simulink library "unifier_obm"  (R2023a)
settings: Solver=VariableStepAuto  StartTime=0.0  StopTime=10.0  RelTol=1e-3
undefined symbols (not defined in the file): b, c, dp_DEP, dp_FUSE_FIN, dp_HTU, dp_VTAIL, dp_VTAIL_INDUCED, dp_WING_root, dp_WING_tip, I, m, S, vtail_nodes, wing_nodes, xyz_cg, xyz_DEP
libraries: sharedutil x7, aerolibtransform2 x4, sharedtransform x2, matrix_library x1, shared6dofsys x1, shared6dof x1, simulink x1
(part 1 of 2)
settings Model: Creator=Thomas  LastModifiedBy=Reggie Johanes
settings DebuggingCC: UnconnectedInputMsg=warning  UnconnectedOutputMsg=warning  UnconnectedLineMsg=warning
settings ModelReferenceCC: EnableRefExpFcnMdlSchedulingChecks=on
settings RTWCC: DLArmComputeVersion=19.05

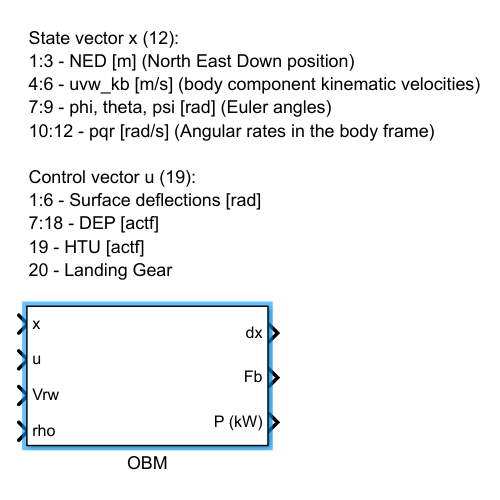
[thumbnail: Simulink's stored preview of the top-level diagram]
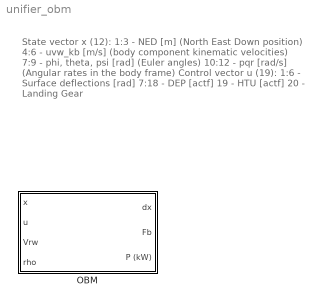
== system unifier_obm ==
  note: State vector x (12):
      | 1:3 - NED [m] (North East Down position)
      | 4:6 - uvw_kb [m/s] (body component kinematic velocities)
      | 7:9 - phi, theta, psi [rad] (Euler angles)
      | 10:12 - pqr [rad/s] (Angular rates in the body frame)
      |
      | Control vector u (19):
      | 1:6 - Surface deflections [rad]
      | 7:18 - DEP [actf]
      | 19 - HTU [actf]
      | 20 - Landing Gear
  OBM : Subsystem

== system unifier_obm/OBM ==
  x : Inport
  u : Inport  Port=2
  Vrw : Inport  Port=3
  rho : Inport  Port=4
  Aero : Subsystem
  Bus Selector : BusSelector  OutputSignals=Vrw,omegarw,Vrw_mag,beta,alpha,rho
  Cast{1,4,6..12} (9 alike) : DataTypeConversion  OutDataTypeStr=single  SaturateOnIntegerOverflow=off  RndMeth=Floor
  Demux : Demux  Outputs=[6,12,1,1]
  EOMandEnviroment : Subsystem
  Subsystems : Subsystem
  Sum : Sum  Inputs=|++
  Sum1 : Sum  Inputs=|++
  dx : Outport
  Fb : Outport  Port=2
  P (kW) : Outport  Port=3
  wires:
  Sum1/1 -> EOMandEnviroment/3(M)
  Cast1/1 -> Aero/8(u1 (rad))
  Subsystems/4(M) -> Sum1/2
  Subsystems/3(F) -> Sum/2
  Subsystems/2(u1_actual) -> Cast1/1
  Sum/1 -> Fb/1, EOMandEnviroment/2(F)
  Cast6/1 -> Aero/7(DEP_J)
  Subsystems/1(DEP_J) -> Cast6/1
  Aero/2(M) -> Sum1/1
  EOMandEnviroment/1(X2) -> Subsystems/1(X2)
  Aero/1(F) -> Sum/1
  u/1 -> Demux/1
  x/1 -> EOMandEnviroment/1(x)
  EOMandEnviroment/3(dx) -> dx/1
  Demux/1 -> Subsystems/3(u1 (rad))  "u1"
  Demux/2 -> Subsystems/4(u2 (actf))  "u2"
  Demux/3 -> Subsystems/5(u3 (actf))  "u3"
  rho/1 -> EOMandEnviroment/4(rho)
  Demux/4 -> Cast4/1  "u4"
  Subsystems/5(P) -> P (kW)/1
  Vrw/1 -> EOMandEnviroment/5(Vrw)
  Bus Selector/4 -> Cast11/1  "<beta>"
  Bus Selector/2 -> Cast9/1  "<omegarw>"
  Cast12/1 -> Aero/5(alpha)
  Bus Selector/6 -> Cast8/1  "<rho>"
  Cast11/1 -> Aero/4(beta)
  Bus Selector/3 -> Cast10/1  "<Vrw_mag>"
  Cast8/1 -> Aero/6(rho)
  Cast7/1 -> Aero/1(Vrw)
  Bus Selector/5 -> Cast12/1  "<alpha>"
  Cast10/1 -> Aero/3(Vrw_mag)
  EOMandEnviroment/2(X4) -> Subsystems/2(X4), Bus Selector/1
  Cast9/1 -> Aero/2(omegarw)
  Bus Selector/1 -> Cast7/1  "<Vrw>"
  Cast4/1 -> Aero/9(u4 (gear))

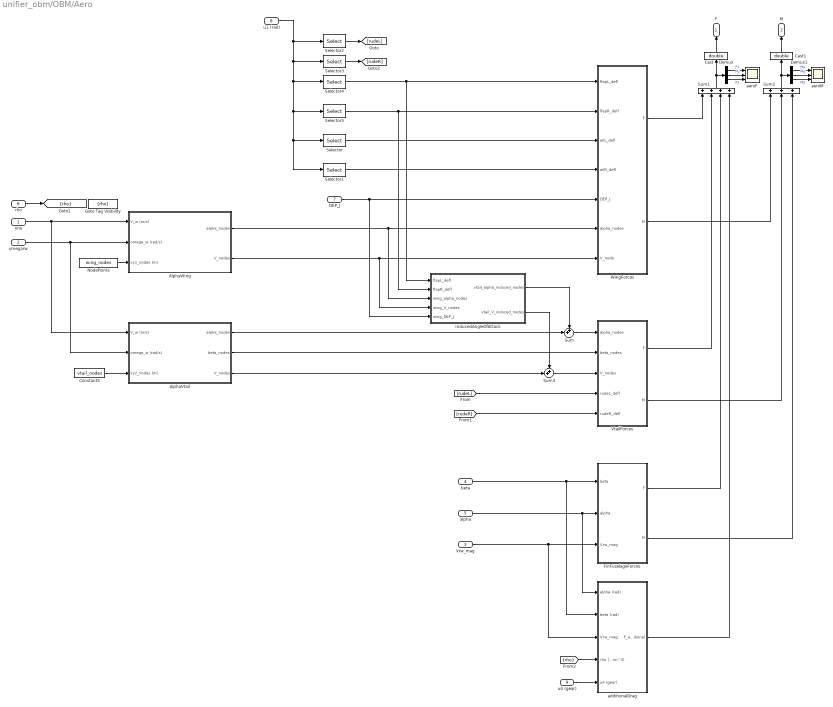
== system unifier_obm/OBM/Aero ==
  Vrw : Inport  OutDataTypeStr=single  Unit=m/s  PortDimensions=3  LockScale=on
  omegarw : Inport  Port=2  OutDataTypeStr=single  Unit=rad/s  PortDimensions=3  LockScale=on
  Vrw_mag : Inport  Port=3  OutDataTypeStr=single
  beta : Inport  Port=4  OutDataTypeStr=single
  alpha : Inport  Port=5  OutDataTypeStr=single
  rho : Inport  Port=6  OutDataTypeStr=single  Unit=kg/m^3  PortDimensions=1  LockScale=on
  DEP_J : Inport  Port=7  OutDataTypeStr=single  PortDimensions=12  LockScale=on
  u1 (rad) : Inport  Port=8
  u4 (gear) : Inport  Port=9
  AlphaVtail : Subsystem  TreatAsAtomicUnit=on
  AlphaWIng : Subsystem  TreatAsAtomicUnit=on
  Cast : DataTypeConversion  OutDataTypeStr=double  SaturateOnIntegerOverflow=off  RndMeth=Floor
  Cast1 : DataTypeConversion  OutDataTypeStr=double  SaturateOnIntegerOverflow=off  RndMeth=Floor
  Constant5 : Constant  Value=vtail_nodes
  Demux : Demux  Outputs=3
  Demux1 : Demux  Outputs=3
  FinFuselageForces : Subsystem
  Goto Tag Visibility : GotoTagVisibility  GotoTag=rho
  InducedAngleOfAttack : Subsystem
  NodePoints : Constant  Value=wing_nodes
  Selector : Selector  InputPortWidth=6  IndexOptions=Index vector (dialog)  Indices=1  OutputSizes=1
  Selector1 : Selector  InputPortWidth=6  IndexOptions=Index vector (dialog)  Indices=2  OutputSizes=1
  Selector2 : Selector  InputPortWidth=6  IndexOptions=Index vector (dialog)  Indices=3  OutputSizes=1
  Selector3 : Selector  InputPortWidth=6  IndexOptions=Index vector (dialog)  Indices=4  OutputSizes=1
  Selector4 : Selector  InputPortWidth=6  IndexOptions=Index vector (dialog)  Indices=5  OutputSizes=1
  Selector5 : Selector  InputPortWidth=6  IndexOptions=Index vector (dialog)  Indices=6  OutputSizes=1
  Sum : Sum  Inputs=++|
  Sum1 : Sum  Inputs=++++
  Sum2 : Sum  Inputs=+++
  Sum3 : Sum  Inputs=++|
  VtailForces : Subsystem
  WingForces : Subsystem
  additionalDrag : Subsystem
  aeroF : Scope  NumInputPorts=3
  aeroM : Scope  NumInputPorts=3
  F : Outport  Unit=N  PortDimensions=3  LockScale=on
  M : Outport  Port=2  Unit=N*m  PortDimensions=3  LockScale=on
  tag scope: rho=scoped
  wires:
  NodePoints/1 -> AlphaWIng/3(xyz_nodes (m))
  Constant5/1 -> AlphaVtail/3(xyz_nodes (m))
  Vrw/1 -> AlphaVtail/1(V_w (m/s)), AlphaWIng/1(V_w (m/s))
  omegarw/1 -> AlphaVtail/2(omega_w (rad/s)), AlphaWIng/2(omega_w (rad/s))
  AlphaWIng/2(V_nodes) -> WingForces/7(V_node), InducedAngleOfAttack/4(wing_V_nodes)
  DEP_J/1 -> WingForces/5(DEP_J), InducedAngleOfAttack/5(wing_DEP_J)
  Sum/1 -> VtailForces/1(alpha_nodes)
  rho/1 -> [rho]
  AlphaVtail/2(beta_nodes) -> VtailForces/2(beta_nodes)
  [rudeL] -> VtailForces/4(rudeL_defl)
  [rudeR] -> VtailForces/5(rudeR_defl)
  WingForces/1(F) -> Sum1/1
  VtailForces/1(F) -> Sum1/2
  WingForces/2(M) -> Sum2/1
  VtailForces/2(M) -> Sum2/2
  Sum1/1 -> Demux/1, Cast/1
  AlphaVtail/3(V_nodes) -> Sum3/2
  InducedAngleOfAttack/1(vtail_alpha_induced_nodes) -> Sum/1
  InducedAngleOfAttack/2(vtail_V_induced_nodes) -> Sum3/1
  Sum3/1 -> VtailForces/3(V_nodes)
  AlphaVtail/1(alpha_nodes) -> Sum/2
  Cast/1 -> F/1
  Cast1/1 -> M/1
  Vrw_mag/1 -> additionalDrag/3(Vrw_mag), FinFuselageForces/3(Vrw_mag)
  beta/1 -> additionalDrag/2(beta (rad)), FinFuselageForces/1(beta)
  FinFuselageForces/1(F) -> Sum1/3
  FinFuselageForces/2(M) -> Sum2/3
  Selector/1 -> WingForces/3(ailL_defl)
  Selector1/1 -> WingForces/4(ailR_defl)
  Selector4/1 -> WingForces/1(flapL_defl), InducedAngleOfAttack/1(flapL_defl)
  Selector5/1 -> WingForces/2(flapR_defl), InducedAngleOfAttack/2(flapR_defl)
  Selector2/1 -> [rudeL]
  Selector3/1 -> [rudeR]
  Demux/1 -> aeroF/1  "Fx"
  Demux/2 -> aeroF/2  "Fy"
  Demux/3 -> aeroF/3  "Fz"
  Sum2/1 -> Cast1/1, Demux1/1
  Demux1/2 -> aeroM/2  "My"
  Demux1/1 -> aeroM/1  "Mx"
  Demux1/3 -> aeroM/3  "Mz"
  AlphaWIng/1(alpha_nodes) -> WingForces/6(alpha_nodes), InducedAngleOfAttack/3(wing_alpha_nodes)
  alpha/1 -> additionalDrag/1(alpha (rad)), FinFuselageForces/2(alpha)
  [rho] -> additionalDrag/4(rho (kg/m^3))
  additionalDrag/1(F_additional) -> Sum1/4
  u4 (gear)/1 -> additionalDrag/5(u4 (gear))
  u1 (rad)/1 -> Selector1/1, Selector/1, Selector5/1, Selector4/1, Selector3/1, Selector2/1

== system unifier_obm/OBM/EOMandEnviroment ==
  note: State vector x (12):
      | 1:3 - NED [m] (North East Down position)
      | 4:6 - uvw_kb [m/s] (body component kinematic velocities)
      | 7:9 - phi, theta, psi [rad] (Euler angles)
      | 10:12 - pqr [rad/s] (Angular rates in the body frame)
  x : Inport
  F : Inport  Port=2
  M : Inport  Port=3
  rho : Inport  Port=4
  Vrw : Inport  Port=5
  Bus Creator : BusCreator  Inputs=8
  Conversion1 : Subsystem
  EOM : Subsystem  mask{mass=m, inertia=I}
      mask prompts: mass "Mass [kg]"; inertia "Inertia [kg/m^3]"
  Mux : Mux  Inputs=2
  Terminator : Terminator
  pqr : Selector  InputPortWidth=12  IndexOptions=Index vector (dialog)  Indices=10:12  OutputSizes=1
  X2 : Outport
  X4 : Outport  Port=2
  dx : Outport  Port=3
  wires:
  Conversion1/3(alpha) -> Bus Creator/5  "alpha"
  Bus Creator/1 -> X4/1
  Conversion1/4(beta) -> Bus Creator/6  "beta"
  Conversion1/1(Vrw_mag) -> Bus Creator/3  "Vrw_mag"
  pqr/1 -> Bus Creator/7, Mux/2  "omegarw"
  EOM/3(DCMbe) -> Bus Creator/1  "DCMbe"
  F/1 -> EOM/2(F)
  M/1 -> EOM/3(M)
  x/1 -> EOM/1(x), pqr/1
  EOM/1(dx) -> dx/1
  rho/1 -> Conversion1/2(rho), Bus Creator/8  "rho"
  Mux/1 -> X2/1
  EOM/2(Abe) -> Terminator/1
  Conversion1/2(Vrw_mag_eas) -> Bus Creator/4  "Vrw_mag_eas"
  Vrw/1 -> Bus Creator/2, Conversion1/1(Vrw), Mux/1  "Vrw"

== system unifier_obm/OBM/Subsystems ==
  X2 : Inport
  X4 : Inport  Port=2
  u1 (rad) : Inport  Port=3
  u2 (actf) : Inport  Port=4
  u3 (actf) : Inport  Port=5
  Actuators : Subsystem
  DEP1 : Subsystem
  Gravity : Subsystem
  HTU : Subsystem
  Sum : Sum  Inputs=+++
  Sum1 : Sum
  Sum2 : Sum  Inputs=|++
  DEP_J : Outport
  u1_actual : Outport  Port=2
  F : Outport  Port=3
  M : Outport  Port=4
  P : Outport  Port=5
  wires:
  X2/1 -> DEP1/1(X2)
  X4/1 -> HTU/2(X4), Gravity/1(X4), DEP1/2(X4)
  DEP1/1(DEP_J) -> DEP_J/1
  Sum/1 -> F/1
  Gravity/1(F) -> Sum/2
  HTU/1(F (N)) -> Sum/3
  Sum1/1 -> M/1
  HTU/2(M (Nm)) -> Sum1/2
  DEP1/2(F) -> Sum/1
  DEP1/3(M) -> Sum1/1
  u1 (rad)/1 -> Actuators/1(u1)
  Actuators/1(u1_actual) -> u1_actual/1
  u3 (actf)/1 -> HTU/1(u3 (actf))
  u2 (actf)/1 -> DEP1/3(u2 (actf))
  DEP1/4(P (kW)) -> Sum2/1
  HTU/3(P (kW)) -> Sum2/2
  Sum2/1 -> P/1

== system unifier_obm/OBM/Aero/AlphaVtail ==
  V_w (m/s) : Inport
  omega_w (rad/s) : Inport  Port=2
  xyz_nodes (m) : Inport  Port=3  Partition=on  PartitionDimension=2  PartitionWidth=1  PartitionOffset=0
  3x3 Cross Product : sharedutil/3x3 Cross Product  aMode=aMode
  Asin : Trigonometry  Operator=asin
  Atan : Trigonometry  Operator=atan
  Cast : DataTypeConversion  OutDataTypeStr=single  SaturateOnIntegerOverflow=off  RndMeth=Floor
  Constant : Constant  Value=xyz_cg
  Constant1 : Constant  Value=eps  OutDataTypeStr=single
  Demux : Demux  Outputs=3
  Divide : Product  Inputs=*/
  Divide1 : Product  Inputs=*/
  For Each : ForEach  DisableCoverage=on  SpecifiedNumIters=16
  Mux : Mux  Inputs=3
  Sum : Sum  Inputs=+-
  Sum1 : Sum  Inputs=++|
  Sum2 : Sum  Inputs=|++
  Sum3 : Sum  Inputs=|++
  V_inf : Fcn  Expr=sqrt(u(1)^2+u(2)^2+u(3)^2)
  alpha_nodes : Outport  ConcatenationDimension=2
  beta_nodes : Outport  Port=2  ConcatenationDimension=2
  V_nodes : Outport  Port=3  ConcatenationDimension=2
  wires:
  3x3 Cross Product/1 -> Sum1/1
  Sum/1 -> 3x3 Cross Product/1
  Constant/1 -> Cast/1
  xyz_nodes (m)/1 -> Sum/2
  omega_w (rad/s)/1 -> 3x3 Cross Product/2
  V_w (m/s)/1 -> Sum1/2
  Sum1/1 -> Demux/1
  Demux/1 -> Sum2/1, Mux/1  "u"
  Demux/3 -> Mux/3, Divide/1  "w"
  Divide/1 -> Atan/1
  Atan/1 -> alpha_nodes/1
  Sum2/1 -> Divide/2
  Constant1/1 -> Sum3/2, Sum2/2
  Divide1/1 -> Asin/1
  Demux/2 -> Mux/2, Divide1/1
  Mux/1 -> V_inf/1
  Asin/1 -> beta_nodes/1  "beta"
  V_inf/1 -> Sum3/1
  Sum3/1 -> V_nodes/1, Divide1/2
  Cast/1 -> Sum/1

== system unifier_obm/OBM/Aero/AlphaWIng ==
  V_w (m/s) : Inport
  omega_w (rad/s) : Inport  Port=2
  xyz_nodes (m) : Inport  Port=3  Partition=on  PartitionDimension=2  PartitionWidth=1  PartitionOffset=0
  Cast : DataTypeConversion  OutDataTypeStr=single  SaturateOnIntegerOverflow=off  RndMeth=Floor
  ComputeAlphaBetaV : Subsystem
  Constant : Constant  Value=xyz_cg
  Cross Product : matrix_library/Cross Product
  For Each : ForEach  DisableCoverage=on  SpecifiedNumIters=14
  Sum : Sum  Inputs=+-
  Sum1 : Sum  Inputs=++|
  Terminator : Terminator
  alpha_nodes : Outport  ConcatenationDimension=2
  V_nodes : Outport  Port=2  ConcatenationDimension=2
  wires:
  Cross Product/1 -> Sum1/1
  Sum/1 -> Cross Product/1
  Constant/1 -> Cast/1
  xyz_nodes (m)/1 -> Sum/2
  omega_w (rad/s)/1 -> Cross Product/2
  V_w (m/s)/1 -> Sum1/2
  Cast/1 -> Sum/1
  Sum1/1 -> ComputeAlphaBetaV/1(V_w_local)
  ComputeAlphaBetaV/3(V_nodes) -> V_nodes/1
  ComputeAlphaBetaV/2(beta_nodes) -> Terminator/1
  ComputeAlphaBetaV/1(alpha_nodes) -> alpha_nodes/1

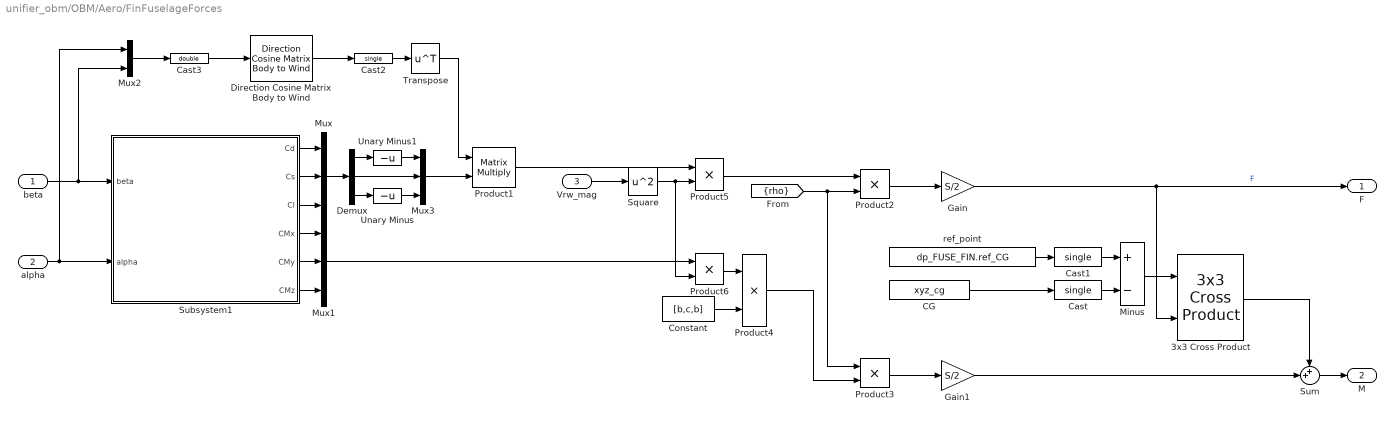
== system unifier_obm/OBM/Aero/FinFuselageForces ==
  beta : Inport
  alpha : Inport  Port=2
  Vrw_mag : Inport  Port=3  OutDataTypeStr=single
  3x3 Cross Product : sharedutil/3x3 Cross Product  aMode=aMode
  CG : Constant  Value=xyz_cg
  Cast : DataTypeConversion  OutDataTypeStr=single  SaturateOnIntegerOverflow=off  RndMeth=Floor
  Cast1 : DataTypeConversion  OutDataTypeStr=single  SaturateOnIntegerOverflow=off  RndMeth=Floor
  Cast2 : DataTypeConversion  OutDataTypeStr=single  SaturateOnIntegerOverflow=off  RndMeth=Floor
  Cast3 : DataTypeConversion  OutDataTypeStr=double  SaturateOnIntegerOverflow=off  RndMeth=Floor
  Constant : Constant  Value=[b,c,b]
  Demux : Demux  Outputs=3
  Direction Cosine Matrix Body to Wind : aerolibtransform2/Direction Cosine Matrix Body to Wind
  Gain : Gain  Gain=S/2
  Gain1 : Gain  Gain=S/2
  Minus : Sum  Inputs=+-
  Mux : Mux  Inputs=3
  Mux1 : Mux  Inputs=3
  Mux2 : Mux  Inputs=2
  Mux3 : Mux  Inputs=3
  Product1 : Product  Multiplication=Matrix(*)
  Product{2..6} (5 alike) : Product
  Square : Math  Operator=square
  Subsystem1 : Subsystem
  Sum : Sum  Inputs=++|
  Transpose : Math  Operator=transpose
  Unary Minus : UnaryMinus
  Unary Minus1 : UnaryMinus
  ref_point : Constant  Value=dp_FUSE_FIN.ref_CG
  F : Outport
  M : Outport  Port=2
  wires:
  Mux/1 -> Demux/1
  Product6/1 -> Product4/1
  Mux1/1 -> Product6/1
  Product5/1 -> Product2/1
  Vrw_mag/1 -> Square/1
  Product1/1 -> Product5/1
  Square/1 -> Product5/2, Product6/2
  Unary Minus1/1 -> Mux3/1
  Unary Minus/1 -> Mux3/3
  Mux3/1 -> Product1/2
  Demux/3 -> Unary Minus/1
  Demux/2 -> Mux3/2
  Demux/1 -> Unary Minus1/1
  Cast2/1 -> Transpose/1
  Cast3/1 -> Direction Cosine Matrix Body to Wind/1
  Direction Cosine Matrix Body to Wind/1 -> Cast2/1
  Transpose/1 -> Product1/1
  Mux2/1 -> Cast3/1
  Sum/1 -> M/1
  alpha/1 -> Subsystem1/2(alpha), Mux2/1
  beta/1 -> Subsystem1/1(beta), Mux2/2
  Cast1/1 -> Minus/1
  CG/1 -> Cast/1
  Minus/1 -> 3x3 Cross Product/1
  Cast/1 -> Minus/2
  ref_point/1 -> Cast1/1
  3x3 Cross Product/1 -> Sum/1
  Subsystem1/6(CMz) -> Mux1/3
  Subsystem1/5(CMy) -> Mux1/2
  Subsystem1/4(CMx) -> Mux1/1
  Subsystem1/3(Cl) -> Mux/3
  Subsystem1/2(Cs) -> Mux/2
  Subsystem1/1(Cd) -> Mux/1
  Product3/1 -> Gain1/1
  Gain/1 -> 3x3 Cross Product/2, F/1  "F"
  Constant/1 -> Product4/2
  [rho] -> Product3/1, Product2/2
  Gain1/1 -> Sum/2
  Product4/1 -> Product3/2
  Product2/1 -> Gain/1

== system unifier_obm/OBM/Aero/InducedAngleOfAttack ==
  flapL_defl : Inport
  flapR_defl : Inport  Port=2
  wing_alpha_nodes : Inport  Port=3  PortDimensions=14
  wing_V_nodes : Inport  Port=4  PortDimensions=14
  wing_DEP_J : Inport  Port=5  PortDimensions=12
  1-D Lookup Table : Lookup_n-D  NumberOfTableDimensions=1  BreakpointsForDimension1=wing_nodes(2,5:10)  BeginIndexSearchUsingPreviousIndexResult=on  TableSource=Input port  Table=tanh([-5:5])  ExtrapMethod=Clip  InternalRulePriority=Speed  RndMeth=Simplest
      settings: InputPortMap=u0,p221
  1-D Lookup Table1 : Lookup_n-D  NumberOfTableDimensions=1  BreakpointsForDimension1=wing_nodes(2,5:10)  BeginIndexSearchUsingPreviousIndexResult=on  TableSource=Input port  Table=tanh([-5:5])  ExtrapMethod=Clip  InternalRulePriority=Speed  RndMeth=Simplest
      settings: InputPortMap=u0,p221
  1-D Lookup Table2 : Lookup_n-D  NumberOfTableDimensions=1  BreakpointsForDimension1=wing_nodes(2,5:10)  BeginIndexSearchUsingPreviousIndexResult=on  TableSource=Input port  Table=tanh([-5:5])  ExtrapMethod=Clip  InternalRulePriority=Speed  RndMeth=Simplest
      settings: InputPortMap=u0,p221
  Constant : Constant  Value=ones(1,8)
  Constant1 : Constant  Value=ones(1,8)
  Constant7 : Constant  Value=vtail_nodes(2,:)
  Mux : Mux  Inputs=2
  Product : Product
  Product1 : Product
  Selector : Selector  InputPortWidth=14  IndexOptions=Index vector (dialog)  Indices=[5:10]  OutputSizes=1
  Selector1 : Selector  InputPortWidth=14  IndexOptions=Index vector (dialog)  Indices=[5:10]  OutputSizes=1
  Selector2 : Selector  InputPortWidth=12  IndexOptions=Index vector (dialog)  Indices=[4:9]  OutputSizes=1
  V_induced : Interpolation_n-D  NumberOfTableDimensions=5  Table=dp_VTAIL_INDUCED.V_induced  NumSelectionDims=1  InternalRulePriority=Speed  TableDataTypeStr=Inherit: Inherit from 'Table data'
      settings: InputPortMap=u0,u1,u2,u3,u4,u5,u6,u7,u8
  alpha_induced : Interpolation_n-D  NumberOfTableDimensions=5  Table=dp_VTAIL_INDUCED.alpha_induced  NumSelectionDims=1  InternalRulePriority=Speed  TableDataTypeStr=Inherit: Inherit from 'Table data'
      settings: InputPortMap=u0,u1,u2,u3,u4,u5,u6,u7,u8
  preLook : Subsystem
  vtail_alpha_induced_nodes : Outport  PortDimensions=16
  vtail_V_induced_nodes : Outport  Port=2  PortDimensions=16
  wires:
  1-D Lookup Table1/1 -> preLook/3(wing_V_inf)
  1-D Lookup Table2/1 -> preLook/4(wing_DEP_J)
  1-D Lookup Table/1 -> preLook/2(wing_alphas)
  Constant7/1 -> 1-D Lookup Table/1, 1-D Lookup Table2/1, 1-D Lookup Table1/1
  wing_V_nodes/1 -> Selector1/1
  wing_alpha_nodes/1 -> Selector/1
  preLook/1(Out1) -> alpha_induced/1, V_induced/1
  preLook/2(Out2) -> alpha_induced/2, V_induced/2
  preLook/3(Out8) -> alpha_induced/3, V_induced/3
  preLook/4(Out9) -> alpha_induced/4, V_induced/4
  preLook/5(Out3) -> alpha_induced/5, V_induced/5
  preLook/6(Out4) -> alpha_induced/6, V_induced/6
  preLook/7(Out6) -> alpha_induced/7, V_induced/7
  preLook/8(Out7) -> alpha_induced/8, V_induced/8
  preLook/9(Out5) -> alpha_induced/9, V_induced/9
  wing_DEP_J/1 -> Selector2/1
  flapL_defl/1 -> Product/2
  Constant/1 -> Product/1
  Constant1/1 -> Product1/1
  flapR_defl/1 -> Product1/2
  Product/1 -> Mux/1
  Product1/1 -> Mux/2
  Mux/1 -> preLook/1(wing_flap_defl)
  V_induced/1 -> vtail_V_induced_nodes/1
  alpha_induced/1 -> vtail_alpha_induced_nodes/1
  Selector/1 -> 1-D Lookup Table/2
  Selector1/1 -> 1-D Lookup Table1/2
  Selector2/1 -> 1-D Lookup Table2/2

== system unifier_obm/OBM/Aero/VtailForces ==
  alpha_nodes : Inport  PortDimensions=16
  beta_nodes : Inport  Port=2  PortDimensions=16
  V_nodes : Inport  Port=3  PortDimensions=16
  rudeL_defl : Inport  Port=4
  rudeR_defl : Inport  Port=5
  Constant : Constant  Value=ones(1,8)
  Constant1 : Constant  Value=ones(1,8)
  Matrix Concatenate1 : Concatenate  NumInputs=3  Mode=Multidimensional array  ConcatenateDimension=2
  Matrix Concatenate2 : Concatenate  NumInputs=3  Mode=Multidimensional array  ConcatenateDimension=2
  Mux : Mux  Inputs=2
  Product : Product
  Product1 : Product
  Reshape : Reshape
  Reshape1 : Reshape
  Subsystem : Subsystem
  Transpose : Math  Operator=transpose
  Transpose1 : Math  Operator=transpose
  VtailForces : Subsystem
  F : Outport
  M : Outport  Port=2
  wires:
  alpha_nodes/1 -> VtailForces/2(alpha_nodes)
  beta_nodes/1 -> VtailForces/3(beta_nodes)
  Product/1 -> Mux/1
  Product1/1 -> Mux/2
  Mux/1 -> VtailForces/1(rude_defl_nodes)
  Constant1/1 -> Product1/1
  Constant/1 -> Product/1
  rudeL_defl/1 -> Product/2
  rudeR_defl/1 -> Product1/2
  VtailForces/4(CMx) -> Matrix Concatenate2/1  "CMx"
  VtailForces/6(CMz) -> Matrix Concatenate2/3  "CMz"
  Matrix Concatenate2/1 -> Transpose1/1
  Subsystem/2(M) -> Reshape/1
  Transpose/1 -> Subsystem/2(F_matrix)
  Transpose1/1 -> Subsystem/3(M_matrix)
  VtailForces/2(Cy) -> Matrix Concatenate1/2  "CFy"
  VtailForces/5(CMy) -> Matrix Concatenate2/2  "CMy"
  VtailForces/1(Cx) -> Matrix Concatenate1/1  "CFx"
  Matrix Concatenate1/1 -> Transpose/1
  Subsystem/1(F) -> Reshape1/1
  VtailForces/3(Cz) -> Matrix Concatenate1/3  "CFz"
  V_nodes/1 -> Subsystem/1(V_nodes)
  Reshape/1 -> M/1
  Reshape1/1 -> F/1

== system unifier_obm/OBM/Aero/WingForces ==
  flapL_defl : Inport
  flapR_defl : Inport  Port=2
  ailL_defl : Inport  Port=3
  ailR_defl : Inport  Port=4
  DEP_J : Inport  Port=5  PortDimensions=12
  alpha_nodes : Inport  Port=6  PortDimensions=14
  V_node : Inport  Port=7  PortDimensions=14
  Demux : Demux  Outputs=3
  Demux1 : Demux  Outputs=3
  Left : Subsystem
  Mux : Mux  Inputs=3
  Mux1 : Mux  Inputs=3
  Reshape : Reshape
  Reshape1 : Reshape
  Right : Subsystem
  Subsystem : Subsystem
  Sum : Sum  Inputs=|++
  Sum1 : Sum  Inputs=|++
  Unary Minus : UnaryMinus
  Unary Minus1 : UnaryMinus
  Unary Minus2 : UnaryMinus
  F : Outport
  M : Outport  Port=2
  wires:
  ailL_defl/1 -> Left/2(aile_defl)
  flapL_defl/1 -> Left/1(flap_defl)
  ailR_defl/1 -> Right/2(aile_defl)
  DEP_J/1 -> Subsystem/1(DEP_J)
  flapR_defl/1 -> Right/1(flap_defl)
  alpha_nodes/1 -> Subsystem/2(alpha_nodes)
  V_node/1 -> Subsystem/3(V_nodes)
  Subsystem/1(DEP_J_Left) -> Left/3(DEP_J)
  Subsystem/2(alpha_nodes_Left) -> Left/4(alpha)
  Subsystem/3(V_nodes_Left) -> Left/5(V_node)
  Left/1(F) -> Demux/1
  Left/2(M) -> Demux1/1
  Demux/2 -> Unary Minus/1
  Demux1/1 -> Unary Minus1/1
  Demux1/3 -> Unary Minus2/1
  Demux1/2 -> Mux/2
  Unary Minus1/1 -> Mux/1
  Unary Minus2/1 -> Mux/3
  Unary Minus/1 -> Mux1/2
  Demux/1 -> Mux1/1
  Demux/3 -> Mux1/3
  Mux1/1 -> Sum/1
  Sum/1 -> F/1
  Mux/1 -> Sum1/1
  Sum1/1 -> M/1
  Right/1(F) -> Reshape/1
  Right/2(M) -> Reshape1/1
  Subsystem/5(alpha_nodes_Right) -> Right/4(alpha)
  Subsystem/6(V_nodes_Right) -> Right/5(V_node)
  Subsystem/4(DEP_J_Right) -> Right/3(DEP_J)
  Reshape/1 -> Sum/2
  Reshape1/1 -> Sum1/2

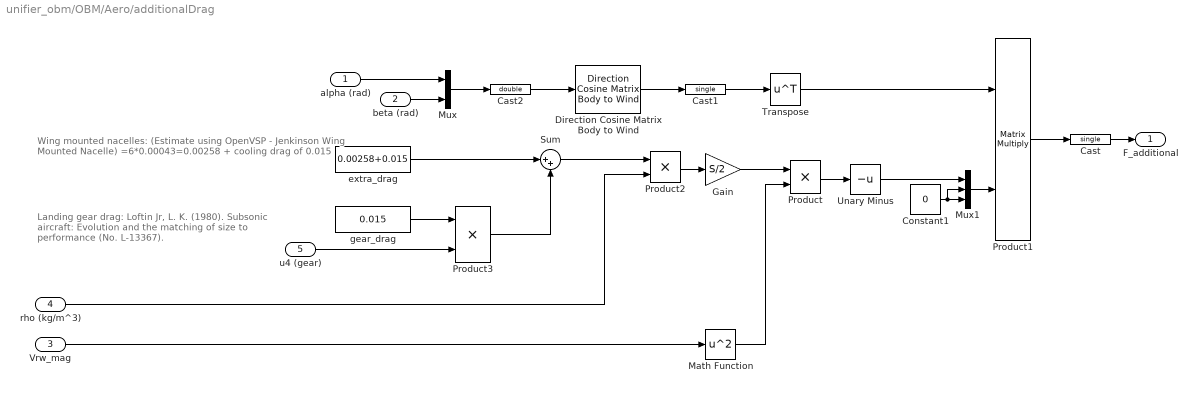
== system unifier_obm/OBM/Aero/additionalDrag ==
  note: Landing gear drag:
      | Loftin Jr, L. K. (1980). Subsonic aircraft: Evolution and the matching of size to performance (No. L-13367).
  note: Wing mounted nacelles:
      | (Estimate using OpenVSP - Jenkinson Wing Mounted Nacelle)
      | =6*0.00043=0.00258
      | + cooling drag of 0.015
  alpha (rad) : Inport
  beta (rad) : Inport  Port=2
  Vrw_mag : Inport  Port=3
  rho (kg/m^3) : Inport  Port=4
  u4 (gear) : Inport  Port=5
  Cast : DataTypeConversion  OutDataTypeStr=single  SaturateOnIntegerOverflow=off  RndMeth=Floor
  Cast1 : DataTypeConversion  OutDataTypeStr=single  SaturateOnIntegerOverflow=off  RndMeth=Floor
  Cast2 : DataTypeConversion  OutDataTypeStr=double  SaturateOnIntegerOverflow=off  RndMeth=Floor
  Constant1 : Constant  Value=0  OutDataTypeStr=single
  Direction Cosine Matrix Body to Wind : aerolibtransform2/Direction Cosine Matrix Body to Wind
  Gain : Gain  Gain=S/2
  Math Function : Math  Operator=square
  Mux : Mux  Inputs=2
  Mux1 : Mux  Inputs=3
  Product : Product  OutDataTypeStr=single
  Product1 : Product  Multiplication=Matrix(*)
  Product2 : Product
  Product3 : Product
  Sum : Sum  Inputs=|++
  Transpose : Math  Operator=transpose
  Unary Minus : UnaryMinus
  extra_drag : Constant  Value=0.00258+0.015  OutDataTypeStr=single
  gear_drag : Constant  Value=0.015  OutDataTypeStr=single
  F_additional : Outport
  wires:
  alpha (rad)/1 -> Mux/1
  Math Function/1 -> Product/2
  Product/1 -> Unary Minus/1
  Gain/1 -> Product/1
  Product2/1 -> Gain/1
  extra_drag/1 -> Sum/1
  Vrw_mag/1 -> Math Function/1
  rho (kg/m^3)/1 -> Product2/2
  Direction Cosine Matrix Body to Wind/1 -> Cast1/1
  Mux/1 -> Cast2/1
  beta (rad)/1 -> Mux/2
  Unary Minus/1 -> Mux1/1
  Transpose/1 -> Product1/1
  Mux1/1 -> Product1/2
  Constant1/1 -> Mux1/2, Mux1/3
  Product1/1 -> Cast/1
  Cast/1 -> F_additional/1
  Cast1/1 -> Transpose/1
  Cast2/1 -> Direction Cosine Matrix Body to Wind/1
  u4 (gear)/1 -> Product3/2
  gear_drag/1 -> Product3/1
  Sum/1 -> Product2/1
  Product3/1 -> Sum/2

== system unifier_obm/OBM/EOMandEnviroment/Conversion1 ==
  Vrw : Inport
  rho : Inport  Port=2
  Add : Sum
  Constant1 : Constant  Value=eps
  Demux3 : Demux  Outputs=3
  Divide1 : Product  Inputs=*/
  Dot Product : DotProduct  OutDataTypeStr=Inherit: Inherit via internal rule
  Gain : Gain  Gain=1/1.225
  Product : Product
  Sqrt : Sqrt
  Sqrt1 : Sqrt
  Trigonometric Function : Trigonometry  Operator=atan2
  Trigonometric Function1 : Trigonometry  Operator=asin
  Vrw_mag : Outport
  Vrw_mag_eas : Outport  Port=2
  alpha : Outport  Port=3
  beta : Outport  Port=4
  wires:
  Demux3/2 -> Divide1/1
  Constant1/1 -> Add/2
  Sqrt/1 -> Add/1
  Divide1/1 -> Trigonometric Function1/1
  Vrw/1 -> Dot Product/1, Dot Product/2, Demux3/1  "V_w"
  Demux3/3 -> Trigonometric Function/1
  Dot Product/1 -> Sqrt/1
  Demux3/1 -> Trigonometric Function/2
  Trigonometric Function1/1 -> beta/1  "beta"
  Trigonometric Function/1 -> alpha/1  "alpha"
  rho/1 -> Gain/1
  Gain/1 -> Sqrt1/1
  Sqrt1/1 -> Product/2
  Product/1 -> Vrw_mag_eas/1
  Add/1 -> Vrw_mag/1, Product/1, Divide1/2

== system unifier_obm/OBM/EOMandEnviroment/EOM ==
  note: Linear acceleration
  note: Euler_dot
  note: pqr_dot
  note: DCM, NED_dot
  x : Inport
  F : Inport  Port=2
  M : Inport  Port=3
  Calculate omega_dot : shared6dofsys/Calculate omega_dot  aMode=aMode
  Constant : Constant  Value=mass
  Constant1 : Constant  Value=inertia
  Constant2 : Constant  Value=zeros(3)
  Demux : Demux  Outputs=[3, 3, 3, 3]
  Mux6 : Mux
  Product : Product  Inputs=*/  SaturateOnIntegerOverflow=on  OutDataTypeStr=Inherit: Same as first input
  Rotation Angles to Direction Cosine Matrix : sharedtransform/Rotation Angles to Direction Cosine Matrix  rotationOrder=ZYX  aMode=aMode
  Selector : Selector  InputPortWidth=3  IndexOptions=Index vector (dialog)  Indices=[3 2 1]  OutputSizes=1
  Subsystem : Subsystem
  Sum : Sum  Inputs=|++  SaturateOnIntegerOverflow=on
  Terminator : Terminator
  Transpose : Math  Operator=transpose  SignedPower=on
  Vbxw : sharedutil/3x3 Cross Product  aMode=aMode
  Vector Concatenate : Concatenate  Mode=Multidimensional array
  "transform to Inertial axes " : shared6dof/6DOF (Euler Angles)/transform to Inertial axes   SystemSampleTime=-1  VariantActivationTime=update diagram  Latency=0  AutoFrameSizeCalculation=off
  dx : Outport
  Abe : Outport  Port=2
  DCMbe : Outport  Port=3
  wires:
  x/1 -> Demux/1
  Transpose/1 -> "transform to Inertial axes "/2
  F/1 -> Product/1
  Vbxw/1 -> Sum/2
  "transform to Inertial axes "/1 -> Mux6/1  "Ve"
  Sum/1 -> Mux6/2  "Abb"
  Product/1 -> Abe/1, Sum/1  "Abe"
  Vector Concatenate/1 -> Calculate omega_dot/2
  M/1 -> Calculate omega_dot/3
  Constant1/1 -> Vector Concatenate/1
  Subsystem/1(phidot thetadot psidot) -> Mux6/3
  Mux6/1 -> dx/1
  Demux/4 -> Subsystem/1(p q r), Calculate omega_dot/1, Vbxw/2  "pqr"
  Rotation Angles to Direction Cosine Matrix/1 -> DCMbe/1, Transpose/1  "DCMbe"
  Constant/1 -> Product/2
  Selector/1 -> Rotation Angles to Direction Cosine Matrix/1
  Demux/3 -> Subsystem/2(phi theta psi), Selector/1  "phithepsi"
  Calculate omega_dot/1 -> Mux6/4
  Constant2/1 -> Vector Concatenate/2
  Demux/2 -> Vbxw/1, "transform to Inertial axes "/1  "uvw_kb"
  Demux/1 -> Terminator/1  "NED"

== system unifier_obm/OBM/Subsystems/Actuators ==
  u1 : Inport
  Demux : Demux  Outputs=6
  Mux : Mux  Inputs=6
  Saturation : Saturate  UpperLimit=deg2rad(25)  LowerLimit=deg2rad(-25)
  Saturation1 : Saturate  UpperLimit=deg2rad(25)  LowerLimit=deg2rad(-25)
  Saturation2 : Saturate  UpperLimit=deg2rad(30)  LowerLimit=deg2rad(-30)
  Saturation3 : Saturate  UpperLimit=deg2rad(30)  LowerLimit=deg2rad(-30)
  Saturation4 : Saturate  UpperLimit=deg2rad(25)  LowerLimit=0
  Saturation6 : Saturate  UpperLimit=deg2rad(25)  LowerLimit=0
  u1_actual : Outport
  wires:
  u1/1 -> Demux/1
  Demux/1 -> Saturation/1
  Demux/2 -> Saturation1/1
  Demux/3 -> Saturation2/1
  Demux/4 -> Saturation3/1
  Saturation3/1 -> Mux/4
  Saturation2/1 -> Mux/3
  Saturation1/1 -> Mux/2
  Saturation/1 -> Mux/1
  Mux/1 -> u1_actual/1
  Demux/5 -> Saturation6/1
  Demux/6 -> Saturation4/1
  Saturation6/1 -> Mux/5
  Saturation4/1 -> Mux/6

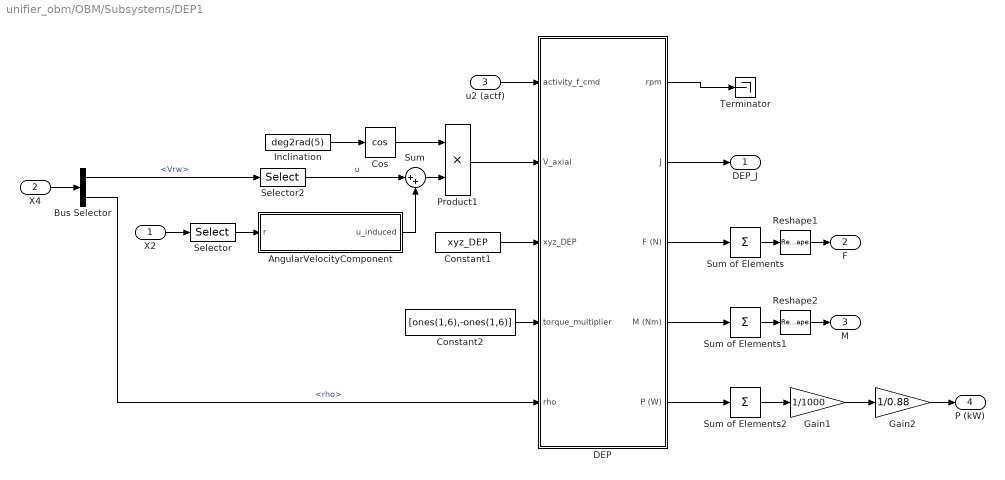
== system unifier_obm/OBM/Subsystems/DEP1 ==
  X2 : Inport
  X4 : Inport  Port=2
  u2 (actf) : Inport  Port=3
  AngularVelocityComponent : Subsystem
  Bus Selector : BusSelector  OutputSignals=Vrw,rho
  Constant1 : Constant  Value=xyz_DEP
  Constant2 : Constant  Value=[ones(1,6),-ones(1,6)]
  Cos : Trigonometry  Operator=cos
  DEP : Subsystem  TreatAsAtomicUnit=on
  Gain1 : Gain  Gain=1/1000
  Gain2 : Gain  Gain=1/0.88
  Inclination : Constant  Value=deg2rad(5)
  Product1 : Product
  Reshape1 : Reshape
  Reshape2 : Reshape
  Selector : Selector  InputPortWidth=6  IndexOptions=Index vector (dialog)  Indices=6  OutputSizes=1
  Selector2 : Selector  InputPortWidth=3  IndexOptions=Index vector (dialog)  Indices=1  OutputSizes=1
  Sum : Sum  Inputs=|++
  Sum of Elements : Sum  Inputs=+  CollapseMode=Specified dimension  CollapseDim=2
  Sum of Elements1 : Sum  Inputs=+  CollapseMode=Specified dimension  CollapseDim=2
  Sum of Elements2 : Sum  Inputs=+  CollapseMode=Specified dimension
  Terminator : Terminator
  DEP_J : Outport
  F : Outport  Port=2
  M : Outport  Port=3
  P (kW) : Outport  Port=4
  wires:
  X2/1 -> Selector/1
  X4/1 -> Bus Selector/1
  Bus Selector/1 -> Selector2/1  "<Vrw>"
  Product1/1 -> DEP/2(V_axial)
  u2 (actf)/1 -> DEP/1(activity_f_cmd)
  DEP/3(F (N)) -> Sum of Elements/1
  DEP/4(M (Nm)) -> Sum of Elements1/1
  Sum of Elements/1 -> Reshape1/1
  Sum of Elements1/1 -> Reshape2/1
  Reshape1/1 -> F/1
  Reshape2/1 -> M/1
  Constant1/1 -> DEP/3(xyz_DEP)
  Constant2/1 -> DEP/4(torque_multiplier)
  Bus Selector/2 -> DEP/5(rho)  "<rho>"
  DEP/2(J) -> DEP_J/1
  DEP/5(P (W)) -> Sum of Elements2/1
  Sum of Elements2/1 -> Gain1/1
  Selector2/1 -> Sum/1  "u"
  Inclination/1 -> Cos/1
  Cos/1 -> Product1/1
  Sum/1 -> Product1/2
  Gain1/1 -> Gain2/1
  Gain2/1 -> P (kW)/1
  Selector/1 -> AngularVelocityComponent/1(r)
  AngularVelocityComponent/1(u_induced) -> Sum/2
  DEP/1(rpm) -> Terminator/1

== system unifier_obm/OBM/Subsystems/Gravity ==
  X4 : Inport
  Bus Selector : BusSelector  OutputSignals=DCMbe
  Constant : Constant  Value=0
  Constant1 : Constant  Value=m
  Multiply : Gain  Gain=9.80665
  Mux : Mux  Inputs=3
  Product : Product  Multiplication=Matrix(*)
  F : Outport
  wires:
  Product/1 -> F/1  "F"
  Bus Selector/1 -> Product/1  "<DCMbe>"
  X4/1 -> Bus Selector/1
  Multiply/1 -> Mux/3
  Constant/1 -> Mux/2, Mux/1
  Mux/1 -> Product/2
  Constant1/1 -> Multiply/1

== system unifier_obm/OBM/Subsystems/HTU ==
  u3 (actf) : Inport
  X4 : Inport  Port=2
  1-D Lookup Table1 : Lookup_n-D  NumberOfTableDimensions=1  BreakpointsForDimension1=[-0.5,1.5]  IndexSearchMethod=Linear search  BeginIndexSearchUsingPreviousIndexResult=on  Table=[-5000, 15000]  ExtrapMethod=Clip  InternalRulePriority=Speed  RndMeth=Simplest
  Bus Selector : BusSelector  OutputSignals=Vrw_mag_eas
  Constant : Constant  Value=0
  Gain : Gain  Gain=1/0.92
  Mux : Mux  Inputs=3
  Mux1 : Mux  Inputs=3
  PropAndMotor : Subsystem
  F (N) : Outport
  M (Nm) : Outport  Port=2
  P (kW) : Outport  Port=3
  wires:
  Mux1/1 -> M (Nm)/1
  Constant/1 -> Mux1/2, Mux1/3, Mux1/1, Mux/3, Mux/2
  Mux/1 -> F (N)/1
  PropAndMotor/2(T (N)) -> Mux/1
  PropAndMotor/1(P (kW)) -> Gain/1
  X4/1 -> Bus Selector/1
  1-D Lookup Table1/1 -> PropAndMotor/2(T_cmd (N))
  Bus Selector/1 -> PropAndMotor/1(Vrw_mag_eas)  "<Vrw_mag_eas>"
  u3 (actf)/1 -> 1-D Lookup Table1/1
  Gain/1 -> P (kW)/1

== system unifier_obm/OBM/Aero/AlphaWIng/ComputeAlphaBetaV ==
  V_w_local : Inport
  Asin : Trigonometry  Operator=asin
  Atan : Trigonometry  Operator=atan
  Constant1 : Constant  Value=eps  OutDataTypeStr=single
  Demux : Demux  Outputs=3
  Divide : Product  Inputs=*/
  Divide1 : Product  Inputs=*/
  Dot Product : DotProduct  OutDataTypeStr=Inherit: Inherit via internal rule
  Square Root : Sqrt
  Sum2 : Sum  Inputs=|++
  alpha_nodes : Outport
  beta_nodes : Outport  Port=2
  V_nodes : Outport  Port=3
  wires:
  V_w_local/1 -> Dot Product/1, Dot Product/2, Demux/1
  Demux/2 -> Divide1/1
  Divide1/1 -> Asin/1
  Demux/1 -> Sum2/1  "u"
  Sum2/1 -> Divide/2
  Square Root/1 -> V_nodes/1, Divide1/2
  Divide/1 -> Atan/1
  Demux/3 -> Divide/1  "w"
  Asin/1 -> beta_nodes/1  "beta"
  Constant1/1 -> Sum2/2
  Dot Product/1 -> Square Root/1
  Atan/1 -> alpha_nodes/1

== system unifier_obm/OBM/Aero/FinFuselageForces/Subsystem1 ==
  beta : Inport
  alpha : Inport  Port=2
  Constant : Constant  Value=0  OutDataTypeStr=single
  Interpolation Using Prelookup : Interpolation_n-D  Table=dp_FUSE_FIN.CD  InternalRulePriority=Speed  TableDataTypeStr=single
  Interpolation Using Prelookup1 : Interpolation_n-D  Table=dp_FUSE_FIN.CS  InternalRulePriority=Speed
  Interpolation Using Prelookup3 : Interpolation_n-D  Table=dp_FUSE_FIN.CMx  InternalRulePriority=Speed
  Interpolation Using Prelookup4 : Interpolation_n-D  Table=dp_FUSE_FIN.CMy  InternalRulePriority=Speed
  Interpolation Using Prelookup5 : Interpolation_n-D  Table=dp_FUSE_FIN.CMz  InternalRulePriority=Speed
  Subsystem : Subsystem
  Cd : Outport
  Cs : Outport  Port=2
  Cl : Outport  Port=3
  CMx : Outport  Port=4
  CMy : Outport  Port=5
  CMz : Outport  Port=6
  wires:
  Interpolation Using Prelookup3/1 -> CMx/1
  Interpolation Using Prelookup/1 -> Cd/1
  Constant/1 -> Cl/1
  Interpolation Using Prelookup5/1 -> CMz/1
  beta/1 -> Subsystem/1(beta)
  Subsystem/3(Out3) -> Interpolation Using Prelookup/3, Interpolation Using Prelookup1/3, Interpolation Using Prelookup3/3, Interpolation Using Prelookup4/3, Interpolation Using Prelookup5/3
  Interpolation Using Prelookup4/1 -> CMy/1
  alpha/1 -> Subsystem/2(alpha)
  Interpolation Using Prelookup1/1 -> Cs/1
  Subsystem/4(Out4) -> Interpolation Using Prelookup/4, Interpolation Using Prelookup1/4, Interpolation Using Prelookup3/4, Interpolation Using Prelookup4/4, Interpolation Using Prelookup5/4
  Subsystem/1(Out1) -> Interpolation Using Prelookup/1, Interpolation Using Prelookup1/1, Interpolation Using Prelookup3/1, Interpolation Using Prelookup4/1, Interpolation Using Prelookup5/1
  Subsystem/2(Out2) -> Interpolation Using Prelookup/2, Interpolation Using Prelookup1/2, Interpolation Using Prelookup3/2, Interpolation Using Prelookup4/2, Interpolation Using Prelookup5/2

== system unifier_obm/OBM/Aero/InducedAngleOfAttack/preLook ==
  wing_flap_defl : Inport
  wing_alphas : Inport  Port=2
  wing_V_inf : Inport  Port=3
  wing_DEP_J : Inport  Port=4
  Constant8 : Constant  Value=0:15
  Prelookup : PreLookup  BreakpointsData=dp_VTAIL_INDUCED.flap_defl  IndexSearchMethod=Linear search  BeginIndexSearchUsingPreviousIndexResult=on  ExtrapMethod=Linear
  Prelookup1 : PreLookup  BreakpointsData=dp_VTAIL_INDUCED.V_infs  IndexSearchMethod=Linear search  BeginIndexSearchUsingPreviousIndexResult=on  ExtrapMethod=Linear
  Prelookup2 : PreLookup  BreakpointsData=dp_VTAIL_INDUCED.alphas  IndexSearchMethod=Linear search  BeginIndexSearchUsingPreviousIndexResult=on  ExtrapMethod=Linear
  Prelookup3 : PreLookup  BreakpointsData=dp_VTAIL_INDUCED.DEP_J  IndexSearchMethod=Linear search  BeginIndexSearchUsingPreviousIndexResult=on
  Out1 : Outport
  Out2 : Outport  Port=2
  Out8 : Outport  Port=3
  Out9 : Outport  Port=4
  Out3 : Outport  Port=5
  Out4 : Outport  Port=6
  Out6 : Outport  Port=7
  Out7 : Outport  Port=8
  Out5 : Outport  Port=9
  wires:
  Prelookup/1 -> Out1/1
  Constant8/1 -> Out5/1
  Prelookup1/2 -> Out4/1
  Prelookup/2 -> Out2/1
  wing_V_inf/1 -> Prelookup1/1
  Prelookup1/1 -> Out3/1
  wing_flap_defl/1 -> Prelookup/1
  wing_alphas/1 -> Prelookup2/1
  wing_DEP_J/1 -> Prelookup3/1
  Prelookup3/1 -> Out6/1
  Prelookup3/2 -> Out7/1
  Prelookup2/1 -> Out8/1
  Prelookup2/2 -> Out9/1

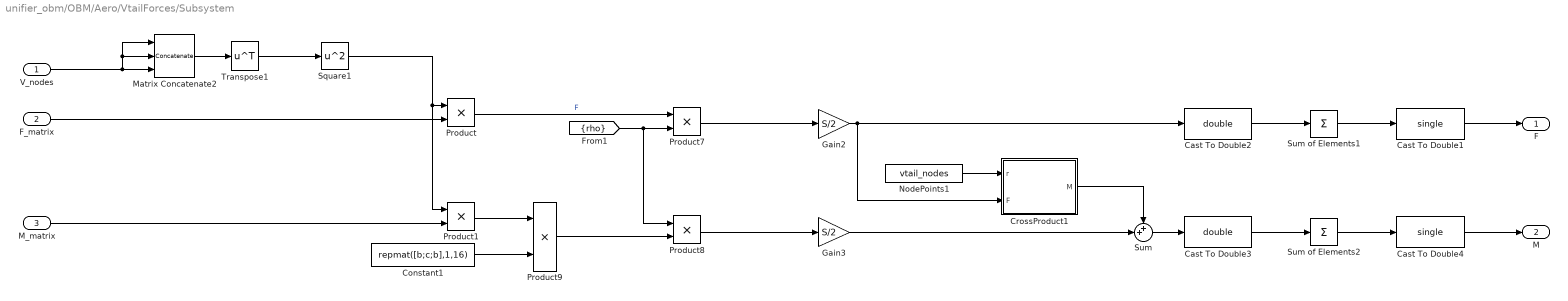
== system unifier_obm/OBM/Aero/VtailForces/Subsystem ==
  V_nodes : Inport
  F_matrix : Inport  Port=2
  M_matrix : Inport  Port=3
  Cast To Double1 : DataTypeConversion  OutDataTypeStr=single  SaturateOnIntegerOverflow=off  RndMeth=Floor
  Cast To Double2 : DataTypeConversion  OutDataTypeStr=double  SaturateOnIntegerOverflow=off  RndMeth=Floor
  Cast To Double3 : DataTypeConversion  OutDataTypeStr=double  SaturateOnIntegerOverflow=off  RndMeth=Floor
  Cast To Double4 : DataTypeConversion  OutDataTypeStr=single  SaturateOnIntegerOverflow=off  RndMeth=Floor
  Constant1 : Constant  Value=repmat([b;c;b],1,16)  VectorParams1D=off  OutDataTypeStr=single
  CrossProduct1 : Subsystem  TreatAsAtomicUnit=on
  Gain2 : Gain  Gain=S/2
  Gain3 : Gain  Gain=S/2
  Matrix Concatenate2 : Concatenate  NumInputs=3  Mode=Multidimensional array  ConcatenateDimension=2
  NodePoints1 : Constant  Value=vtail_nodes
  Product{,1,7..9} (5 alike) : Product
  Square1 : Math  Operator=square
  Sum : Sum  Inputs=++|
  Sum of Elements1 : Sum  Inputs=+  CollapseMode=Specified dimension  CollapseDim=2
  Sum of Elements2 : Sum  Inputs=+  CollapseMode=Specified dimension  CollapseDim=2
  Transpose1 : Math  Operator=transpose
  F : Outport
  M : Outport  Port=2
  wires:
  Sum/1 -> Cast To Double3/1
  Gain2/1 -> CrossProduct1/2(F), Cast To Double2/1
  Sum of Elements2/1 -> Cast To Double4/1
  Sum of Elements1/1 -> Cast To Double1/1
  Transpose1/1 -> Square1/1
  Product/1 -> Product7/1  "F"
  Product7/1 -> Gain2/1
  Square1/1 -> Product1/1, Product/1
  Matrix Concatenate2/1 -> Transpose1/1
  Gain3/1 -> Sum/2
  Product9/1 -> Product8/2
  NodePoints1/1 -> CrossProduct1/1(r)
  [rho] -> Product8/1, Product7/2
  Product8/1 -> Gain3/1
  Constant1/1 -> Product9/2
  M_matrix/1 -> Product1/2
  Product1/1 -> Product9/1
  CrossProduct1/1(M) -> Sum/1
  F_matrix/1 -> Product/2
  V_nodes/1 -> Matrix Concatenate2/1, Matrix Concatenate2/2, Matrix Concatenate2/3
  Cast To Double2/1 -> Sum of Elements1/1
  Cast To Double1/1 -> F/1
  Cast To Double3/1 -> Sum of Elements2/1
  Cast To Double4/1 -> M/1

== system unifier_obm/OBM/Aero/VtailForces/VtailForces ==
  rude_defl_nodes : Inport
  alpha_nodes : Inport  Port=2
  beta_nodes : Inport  Port=3
  Interpolation Using Prelookup1 : Interpolation_n-D  NumberOfTableDimensions=4  Table=dp_VTAIL.CFx  NumSelectionDims=1  InternalRulePriority=Speed  TableDataTypeStr=Inherit: Inherit from 'Table data'
      settings: InputPortMap=u0,u1,u2,u3,u4,u5,u6
  Interpolation Using Prelookup2 : Interpolation_n-D  NumberOfTableDimensions=4  Table=dp_VTAIL.CFy  NumSelectionDims=1  InternalRulePriority=Speed  TableDataTypeStr=Inherit: Inherit from 'Table data'
      settings: InputPortMap=u0,u1,u2,u3,u4,u5,u6
  Interpolation Using Prelookup3 : Interpolation_n-D  NumberOfTableDimensions=4  Table=dp_VTAIL.CFz  NumSelectionDims=1  InternalRulePriority=Speed  TableDataTypeStr=Inherit: Inherit from 'Table data'
      settings: InputPortMap=u0,u1,u2,u3,u4,u5,u6
  Interpolation Using Prelookup4 : Interpolation_n-D  NumberOfTableDimensions=4  Table=dp_VTAIL.CMx  NumSelectionDims=1  InternalRulePriority=Speed  TableDataTypeStr=Inherit: Inherit from 'Table data'
      settings: InputPortMap=u0,u1,u2,u3,u4,u5,u6
  Interpolation Using Prelookup5 : Interpolation_n-D  NumberOfTableDimensions=4  Table=dp_VTAIL.CMy  NumSelectionDims=1  InternalRulePriority=Speed  TableDataTypeStr=Inherit: Inherit from 'Table data'
      settings: InputPortMap=u0,u1,u2,u3,u4,u5,u6
  Interpolation Using Prelookup6 : Interpolation_n-D  NumberOfTableDimensions=4  Table=dp_VTAIL.CMz  NumSelectionDims=1  InternalRulePriority=Speed  TableDataTypeStr=Inherit: Inherit from 'Table data'
      settings: InputPortMap=u0,u1,u2,u3,u4,u5,u6
  WingRootPreLookup : Subsystem
  Cx : Outport
  Cy : Outport  Port=2
  Cz : Outport  Port=3
  CMx : Outport  Port=4
  CMy : Outport  Port=5
  CMz : Outport  Port=6
  wires:
  WingRootPreLookup/3(Out3) -> Interpolation Using Prelookup2/3, Interpolation Using Prelookup6/3, Interpolation Using Prelookup5/3, Interpolation Using Prelookup4/3, Interpolation Using Prelookup3/3, Interpolation Using Prelookup1/3
  rude_defl_nodes/1 -> WingRootPreLookup/1(rude_defl_nodes)
  WingRootPreLookup/4(Out4) -> Interpolation Using Prelookup6/4, Interpolation Using Prelookup5/4, Interpolation Using Prelookup4/4, Interpolation Using Prelookup3/4, Interpolation Using Prelookup2/4, Interpolation Using Prelookup1/4
  WingRootPreLookup/5(Out6) -> Interpolation Using Prelookup4/5, Interpolation Using Prelookup6/5, Interpolation Using Prelookup5/5, Interpolation Using Prelookup3/5, Interpolation Using Prelookup2/5, Interpolation Using Prelookup1/5
  Interpolation Using Prelookup1/1 -> Cx/1
  WingRootPreLookup/6(Out7) -> Interpolation Using Prelookup6/6, Interpolation Using Prelookup5/6, Interpolation Using Prelookup4/6, Interpolation Using Prelookup3/6, Interpolation Using Prelookup2/6, Interpolation Using Prelookup1/6
  WingRootPreLookup/2(Out2) -> Interpolation Using Prelookup4/2, Interpolation Using Prelookup5/2, Interpolation Using Prelookup6/2, Interpolation Using Prelookup3/2, Interpolation Using Prelookup2/2, Interpolation Using Prelookup1/2
  beta_nodes/1 -> WingRootPreLookup/3(beta_nodes)
  alpha_nodes/1 -> WingRootPreLookup/2(alpha_nodes)
  WingRootPreLookup/7(Out5) -> Interpolation Using Prelookup5/7, Interpolation Using Prelookup6/7, Interpolation Using Prelookup4/7, Interpolation Using Prelookup3/7, Interpolation Using Prelookup2/7, Interpolation Using Prelookup1/7
  Interpolation Using Prelookup2/1 -> Cy/1
  Interpolation Using Prelookup3/1 -> Cz/1
  Interpolation Using Prelookup4/1 -> CMx/1
  Interpolation Using Prelookup5/1 -> CMy/1
  Interpolation Using Prelookup6/1 -> CMz/1
  WingRootPreLookup/1(Out1) -> Interpolation Using Prelookup6/1, Interpolation Using Prelookup5/1, Interpolation Using Prelookup4/1, Interpolation Using Prelookup3/1, Interpolation Using Prelookup2/1, Interpolation Using Prelookup1/1

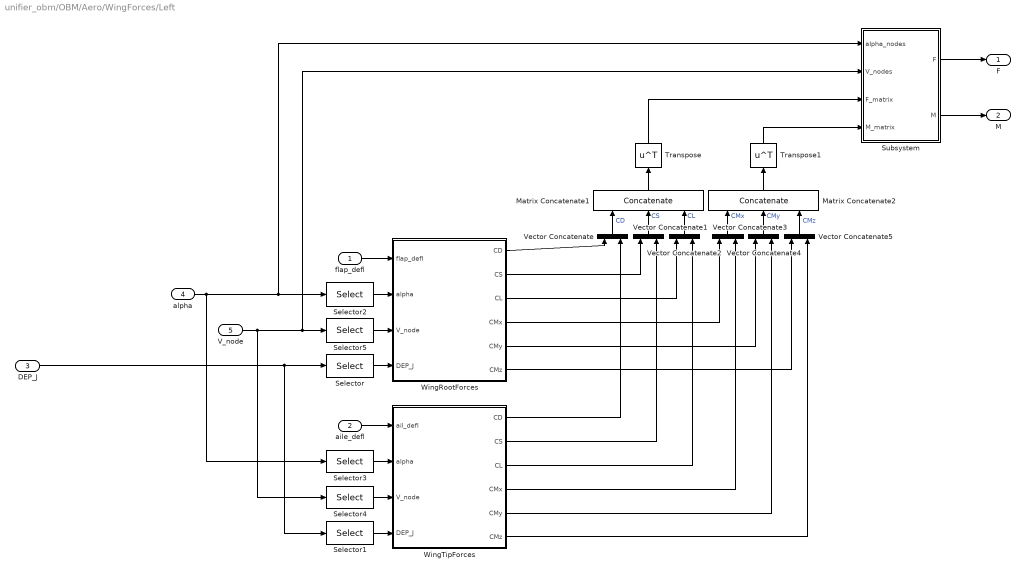
== system unifier_obm/OBM/Aero/WingForces/Left ==
  flap_defl : Inport
  aile_defl : Inport  Port=2
  DEP_J : Inport  Port=3  PortDimensions=6
  alpha : Inport  Port=4  PortDimensions=7
  V_node : Inport  Port=5  PortDimensions=7
  Matrix Concatenate1 : Concatenate  NumInputs=3  Mode=Multidimensional array  ConcatenateDimension=2
  Matrix Concatenate2 : Concatenate  NumInputs=3  Mode=Multidimensional array  ConcatenateDimension=2
  Selector : Selector  InputPortWidth=6  IndexOptions=Index vector (dialog)  Indices=[1,2,3,4,5]  OutputSizes=1
  Selector1 : Selector  InputPortWidth=6  IndexOptions=Index vector (dialog)  Indices=[5,6]  OutputSizes=1
  Selector2 : Selector  InputPortWidth=7  IndexOptions=Index vector (dialog)  Indices=[1,2,3,4,5]  OutputSizes=1
  Selector3 : Selector  InputPortWidth=7  IndexOptions=Index vector (dialog)  Indices=[6,7]  OutputSizes=1
  Selector4 : Selector  InputPortWidth=7  IndexOptions=Index vector (dialog)  Indices=[6,7]  OutputSizes=1
  Selector5 : Selector  InputPortWidth=7  IndexOptions=Index vector (dialog)  Indices=[1,2,3,4,5]  OutputSizes=1
  Subsystem : Subsystem
  Transpose : Math  Operator=transpose
  Transpose1 : Math  Operator=transpose
  Vector Concatenate{,1..5} (6 alike) : Concatenate
  WingRootForces : Subsystem
  WingTipForces : Subsystem
  F : Outport
  M : Outport  Port=2
  wires:
  flap_defl/1 -> WingRootForces/1(flap_defl)
  alpha/1 -> Subsystem/1(alpha_nodes), Selector2/1, Selector3/1
  DEP_J/1 -> Selector1/1, Selector/1
  Selector/1 -> WingRootForces/4(DEP_J)
  V_node/1 -> Selector4/1, Subsystem/2(V_nodes), Selector5/1
  WingRootForces/1(CD) -> Vector Concatenate/1
  Selector1/1 -> WingTipForces/4(DEP_J)
  WingRootForces/6(CMz) -> Vector Concatenate5/1
  WingTipForces/1(CD) -> Vector Concatenate/2
  WingTipForces/6(CMz) -> Vector Concatenate5/2
  WingTipForces/2(CS) -> Vector Concatenate1/2
  WingTipForces/3(CL) -> Vector Concatenate2/2
  WingTipForces/5(CMy) -> Vector Concatenate4/2
  WingTipForces/4(CMx) -> Vector Concatenate3/2
  aile_defl/1 -> WingTipForces/1(ail_defl)
  Selector2/1 -> WingRootForces/2(alpha)
  Selector3/1 -> WingTipForces/2(alpha)
  Selector4/1 -> WingTipForces/3(V_node)
  Selector5/1 -> WingRootForces/3(V_node)
  WingRootForces/2(CS) -> Vector Concatenate1/1
  WingRootForces/3(CL) -> Vector Concatenate2/1
  WingRootForces/4(CMx) -> Vector Concatenate3/1
  WingRootForces/5(CMy) -> Vector Concatenate4/1
  Vector Concatenate1/1 -> Matrix Concatenate1/2  "CS"
  Matrix Concatenate1/1 -> Transpose/1
  Vector Concatenate/1 -> Matrix Concatenate1/1  "CD"
  Vector Concatenate2/1 -> Matrix Concatenate1/3  "CL"
  Vector Concatenate3/1 -> Matrix Concatenate2/1  "CMx"
  Vector Concatenate4/1 -> Matrix Concatenate2/2  "CMy"
  Vector Concatenate5/1 -> Matrix Concatenate2/3  "CMz"
  Matrix Concatenate2/1 -> Transpose1/1
  Transpose/1 -> Subsystem/3(F_matrix)
  Transpose1/1 -> Subsystem/4(M_matrix)
  Subsystem/1(F) -> F/1
  Subsystem/2(M) -> M/1

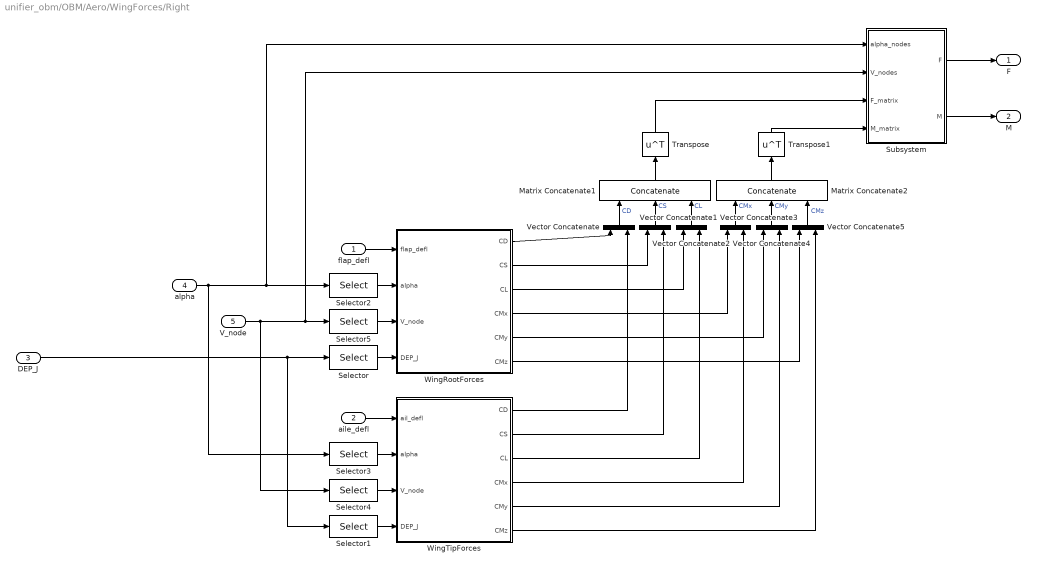
== system unifier_obm/OBM/Aero/WingForces/Right ==
  flap_defl : Inport
  aile_defl : Inport  Port=2
  DEP_J : Inport  Port=3  PortDimensions=6
  alpha : Inport  Port=4  PortDimensions=7
  V_node : Inport  Port=5  PortDimensions=7
  Matrix Concatenate1 : Concatenate  NumInputs=3  Mode=Multidimensional array  ConcatenateDimension=2
  Matrix Concatenate2 : Concatenate  NumInputs=3  Mode=Multidimensional array  ConcatenateDimension=2
  Selector : Selector  InputPortWidth=6  IndexOptions=Index vector (dialog)  Indices=[1,2,3,4,5]  OutputSizes=1
  Selector1 : Selector  InputPortWidth=6  IndexOptions=Index vector (dialog)  Indices=[5,6]  OutputSizes=1
  Selector2 : Selector  InputPortWidth=7  IndexOptions=Index vector (dialog)  Indices=[1,2,3,4,5]  OutputSizes=1
  Selector3 : Selector  InputPortWidth=7  IndexOptions=Index vector (dialog)  Indices=[6,7]  OutputSizes=1
  Selector4 : Selector  InputPortWidth=7  IndexOptions=Index vector (dialog)  Indices=[6,7]  OutputSizes=1
  Selector5 : Selector  InputPortWidth=7  IndexOptions=Index vector (dialog)  Indices=[1,2,3,4,5]  OutputSizes=1
  Subsystem : Subsystem
  Transpose : Math  Operator=transpose
  Transpose1 : Math  Operator=transpose
  Vector Concatenate{,1..5} (6 alike) : Concatenate
  WingRootForces : Subsystem
  WingTipForces : Subsystem
  F : Outport
  M : Outport  Port=2
  wires:
  flap_defl/1 -> WingRootForces/1(flap_defl)
  alpha/1 -> Subsystem/1(alpha_nodes), Selector2/1, Selector3/1
  DEP_J/1 -> Selector1/1, Selector/1
  Selector/1 -> WingRootForces/4(DEP_J)
  V_node/1 -> Selector4/1, Subsystem/2(V_nodes), Selector5/1
  WingRootForces/1(CD) -> Vector Concatenate/1
  Selector1/1 -> WingTipForces/4(DEP_J)
  WingRootForces/6(CMz) -> Vector Concatenate5/1
  WingTipForces/1(CD) -> Vector Concatenate/2
  WingTipForces/6(CMz) -> Vector Concatenate5/2
  WingTipForces/2(CS) -> Vector Concatenate1/2
  WingTipForces/3(CL) -> Vector Concatenate2/2
  WingTipForces/5(CMy) -> Vector Concatenate4/2
  WingTipForces/4(CMx) -> Vector Concatenate3/2
  aile_defl/1 -> WingTipForces/1(ail_defl)
  Selector2/1 -> WingRootForces/2(alpha)
  Selector3/1 -> WingTipForces/2(alpha)
  Selector4/1 -> WingTipForces/3(V_node)
  Selector5/1 -> WingRootForces/3(V_node)
  WingRootForces/2(CS) -> Vector Concatenate1/1
  WingRootForces/3(CL) -> Vector Concatenate2/1
  WingRootForces/4(CMx) -> Vector Concatenate3/1
  WingRootForces/5(CMy) -> Vector Concatenate4/1
  Vector Concatenate1/1 -> Matrix Concatenate1/2  "CS"
  Matrix Concatenate1/1 -> Transpose/1
  Vector Concatenate/1 -> Matrix Concatenate1/1  "CD"
  Vector Concatenate2/1 -> Matrix Concatenate1/3  "CL"
  Vector Concatenate3/1 -> Matrix Concatenate2/1  "CMx"
  Vector Concatenate4/1 -> Matrix Concatenate2/2  "CMy"
  Vector Concatenate5/1 -> Matrix Concatenate2/3  "CMz"
  Matrix Concatenate2/1 -> Transpose1/1
  Transpose/1 -> Subsystem/3(F_matrix)
  Transpose1/1 -> Subsystem/4(M_matrix)
  Subsystem/1(F) -> F/1
  Subsystem/2(M) -> M/1

== system unifier_obm/OBM/Aero/WingForces/Subsystem ==
  DEP_J : Inport
  alpha_nodes : Inport  Port=2
  V_nodes : Inport  Port=3
  Demux1 : Demux  Outputs=2
  Demux2 : Demux  Outputs=2
  Demux3 : Demux  Outputs=2
  Selector : Selector  InputPortWidth=6  IndexOptions=Index vector (dialog)  Indices=[6,5,4,3,2,1]  OutputSizes=1
  Selector1 : Selector  InputPortWidth=7  IndexOptions=Index vector (dialog)  Indices=[7,6,5,4,3,2,1]  OutputSizes=1
  Selector2 : Selector  InputPortWidth=7  IndexOptions=Index vector (dialog)  Indices=[7,6,5,4,3,2,1]  OutputSizes=1
  DEP_J_Left : Outport  PortDimensions=6
  alpha_nodes_Left : Outport  Port=2  PortDimensions=7
  V_nodes_Left : Outport  Port=3  PortDimensions=7
  DEP_J_Right : Outport  Port=4  PortDimensions=6
  alpha_nodes_Right : Outport  Port=5  PortDimensions=7
  V_nodes_Right : Outport  Port=6  PortDimensions=7
  wires:
  Demux2/2 -> DEP_J_Right/1
  Demux2/1 -> Selector/1
  DEP_J/1 -> Demux2/1
  Selector/1 -> DEP_J_Left/1
  Selector1/1 -> alpha_nodes_Left/1
  alpha_nodes/1 -> Demux1/1
  Demux1/2 -> alpha_nodes_Right/1
  Demux1/1 -> Selector1/1
  Demux3/1 -> Selector2/1
  Selector2/1 -> V_nodes_Left/1
  V_nodes/1 -> Demux3/1
  Demux3/2 -> V_nodes_Right/1

== system unifier_obm/OBM/EOMandEnviroment/EOM/Subsystem ==
  p q r : Inport
  phi theta psi : Inport  Port=2
  Mux1 : Mux  Inputs=[3 3 3]
  Mux2 : Mux  Inputs=3
  phidot : Fcn  Expr=u[1]+(u[2]*u[4]+u[3]*u[7])*(u[5]/u[8])
  psidot : Fcn  Expr=(u[2]*u[4]+u[3]*u[7])/u[8]
  sincos : Trigonometry  Operator=sincos
  thetadot : Fcn  Expr=u[2]*u[7]-u[3]*u[4]
  phidot thetadot psidot : Outport  InitialOutput=0  VectorParamsAs1DForOutWhenUnconnected=off
  wires:
  Mux1/1 -> psidot/1, phidot/1, thetadot/1
  sincos/1 -> Mux1/2
  psidot/1 -> Mux2/3
  thetadot/1 -> Mux2/2
  p q r/1 -> Mux1/1
  Mux2/1 -> phidot thetadot psidot/1
  phidot/1 -> Mux2/1
  phi theta psi/1 -> sincos/1
  sincos/2 -> Mux1/3

== system unifier_obm/OBM/Subsystems/DEP1/AngularVelocityComponent ==
  r : Inport
  Constant : Constant  Value=xyz_DEP
  Constant4 : Constant  Value=xyz_cg
  Gain : Gain  Gain=ones(1,12)
  Product : Product
  Reshape : Reshape
  Reshape3 : Reshape
  Selector1 : Selector  NumberOfDimensions=2  InputPortWidth=6  IndexOptions=Index vector (dialog),Select all  Indices=2,1  OutputSizes=1,1
  Selector3 : Selector  InputPortWidth=3  IndexOptions=Index vector (dialog)  Indices=2  OutputSizes=1
  Sum1 : Sum  Inputs=|+-
  u_induced : Outport
  wires:
  Selector1/1 -> Reshape/1
  Constant4/1 -> Selector3/1
  Sum1/1 -> Product/2
  Selector3/1 -> Gain/1
  Gain/1 -> Reshape3/1
  Reshape3/1 -> Sum1/1
  r/1 -> Product/1
  Constant/1 -> Selector1/1
  Reshape/1 -> Sum1/2
  Product/1 -> u_induced/1
